simulink model "PEMFuelCellSystem_Before_v01"  (R2025b)
settings: Solver=VariableStepAuto  StartTime=0.0  StopTime=0.1  MaxStep=0.01  RelTol=1e-3  AbsTol=1e-3
model workspace: external: MATLAB File E:\agentwork_pemfc_cEGR_0519\04_Simulink物理网络模型\01_模型\RouteA_GasMixture_Derived\PEMFuelCellSystemWithACustomLibraryParameters.m (data not in the file)
undefined symbols (not defined in the file): anode_tube_D, cathode_tube_D, cegr_valve_max_area, cegr_valve_open_min_area, comp_rpm_TLU, coolant_num_layers, coolant_num_passes, coolant_tube_D, coolant_w_channels, env_p, env_T, env_yH20, env_yO2, radiator_air_area_fins, radiator_air_area_primary, radiator_eta_fin, radiator_N_tubes, radiator_rho, radiator_t_wall, radiator_tube_H, radiator_W, routeA_air_pid_Ki, routeA_air_pid_Kp, routeA_anode_inlet_pressure_MPa_abs, routeA_anode_purge_off_n2_mole_fraction, routeA_anode_purge_on_n2_mole_fraction, routeA_anode_recirculation_base_command, routeA_anode_recirculation_current_gain_A_inv, routeA_anode_rh_setpoint, routeA_cathode_humidifier_gain, routeA_cathode_rh_setpoint, routeA_compressor_cmd_direct, routeA_egr_control_Ki_area, routeA_egr_control_Kp_area, routeA_egr_target_input_mode_id, routeA_egr_valve_actuator_tau, routeA_egr_valve_area_direct, routeA_stack_temperature_set_C, routeA_target_egr_ratio_comp_in, routeA_target_mdot_comp_inlet, routeA_target_oer, routeA_target_p_ca_out_MPa, routeA_voltage_current_max_A, routeA_voltage_current_min_A, routeA_voltage_pi_Ki, routeA_voltage_pi_Kp, stack_area, stack_iL, stack_mea_rho, stack_num_cells, stack_num_channels, stack_t_gdl, stack_t_membrane, stack_w_channels, tank_yH2
libraries: fl_lib x63, FuelCell_lib x53, nesl_utility x42, slpidlib x5
(part 1 of 6)
CloseFcn:
  | try,close(h1_PEMFuelCellSystemWithACustomLibrary),end
  | clear h1_PEMFuelCellSystemWithACustomLibrary
  | try,close(h2_PEMFuelCellSystemWithACustomLibrary),end
  | clear h2_PEMFuelCellSystemWithACustomLibrary
  | try,close(h3_PEMFuelCellSystemWithACustomLibrary),end
  | clear h3_PEMFuelCellSystemWithACustomLibrary
  | try,close(h4_PEMFuelCellSystemWithACustomLibrary),end
  | clear h4_PEMFuelCellSystemWithACustomLibrary
  | try,close(h5_PEMFuelCellSystemWithACustomLibrary),end
  | clear h5_PEMFuelCellSystemWithACustomLibrary
  | try,close(h6_PEMFuelCellSystemWithACustomLibrary),end
  | clear h6_PEMFuelCellSystemWithACustomLibrary
  | 
  | clear tout simlog_PEMFuelCellSystemWithACustomLibrary
Description:
  | PEM Fuel Cell System with a Custom Library
settings Model: Creator=The MathWorks, Inc.  LastModifiedBy=ADMIN
settings SolverCC: AutoScaleAbsTol=off  MaxConsecutiveMinStep=10  AlgebraicLoopSolver=TrustRegion  MaxZcPerStep=1.0
settings DataIOCC: SaveFormat=Array  ReturnWorkspaceOutputs=off
settings DebuggingCC: UnconnectedInputMsg=warning  UnconnectedOutputMsg=warning  UnconnectedLineMsg=warning  SymbolicDimsDataTypeCodeGenerationDiagnostic=none
settings ModelReferenceCC: EnableRefExpFcnMdlSchedulingChecks=on
settings SFSimCC: CustomCodeUndefinedFunction=UseInterfaceOnly
settings RTWCC: GPUComputeCapability=3.5  DLArmComputeVersion=19.05
settings SimscapeCC: SimscapeLogType=all  SimscapeLogSimulationStatistics=on  SimscapeLogName=simlog_PEMFuelCellSystem_GasMixture_cEGR_RouteA_v01  SimscapeLogDataHistory=20000.0

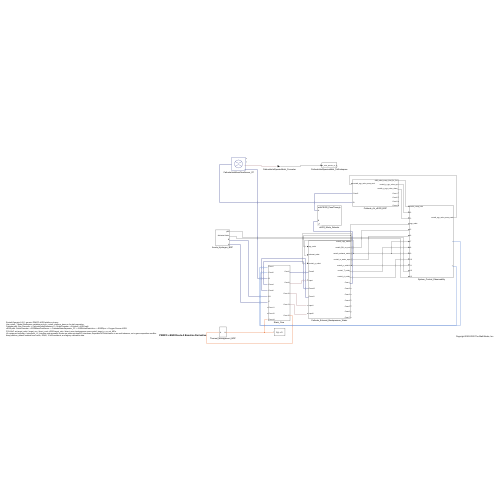
[thumbnail: Simulink's stored preview of the top-level diagram]
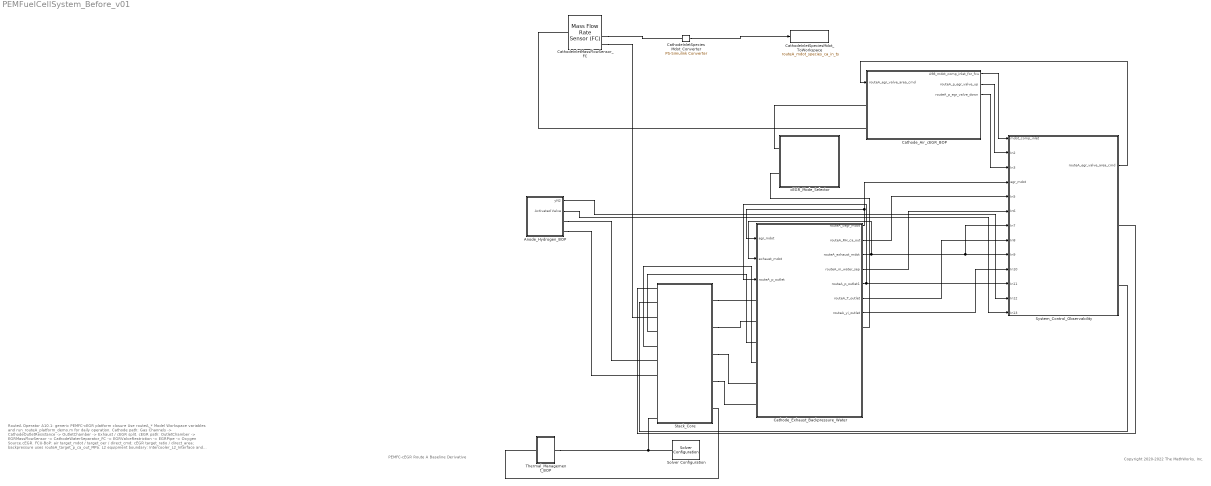
== system PEMFuelCellSystem_Before_v01 ==
  note: PEMFC-cEGR Route A Baseline Derivative
  note: RouteA Operator A10.1: generic PEMFC-cEGR platform closure
      | Use routeA_* Model Workspace variables and run_routeA_platform_demo.m for daily operation.
      | Cathode path: Gas Channels -> CathodeOutletResistance -> OutletChamber -> Exhaust / cEGR split.
      | cEGR path: OutletChamber -> EGRMassFlowSensor -> CathodeWaterSeparator_FC -> EGRValveRestriction -> EGRPipe -> Oxygen Source.cEGR.
      | FCU-BoP: air target_mdot / target_oer / direct_cmd; cEGR target_ratio / direct_area; backpressure uses routeA_target_p_ca_out_MPa.
      | L2 equipment boundary: Intercooler_L2_Interface and separator blocks are pressure-drop/KPI interfaces; SeparatorOrCondensation is an audit observer, not a gas-composition modifier.
      | Keep platform_default isolated from bench, DQ60, 10 kW workbook, and legacy calibration data.
  note: Copyright 2020-2022 The MathWorks, Inc.
  Anode_Hydrogen_BOP : Subsystem
  CathodeInletMassFlowSensor_FC : FuelCell_lib/sensors/Mass Flow Rate Sensor (FC)
      settings: InternalSimscapePortConfiguration="{\"Bottom\":[],\"Left\":[{\"id\":\"A\",\"label\":\"A\",\"type\":\"FuelCell.FuelCell\"}],\"Right\":[{\"id\":\"M\",\"label\":\"M\",\"type\":\"output\"},{\"id\":\"Phi_out\",\"label\":\"Phi\",\"type\":\"output\"},{\"id\":\"M_i\",\"label\":\"M_i\",\"type\":\"output\"},{\"id\":\"B\",\"label\":\"B\",\"type\":\"FuelCell.FuelCell\"}],\"Top\":[]}"
  CathodeInletSpeciesMdot_Converter : nesl_utility/PS-Simulink Converter  PhysicalDomain=network_engine_domain  SubClassName=ps_output  LeftPortType=input  RightPortType=output  PseudoPeriodic=off  Frequencies=[]  VectorFormat=inherit  Unit=inherit  AffineConversion=off
  CathodeInletSpeciesMdot_ToWorkspace : ToWorkspace  VariableName=routeA_mdot_species_ca_in_ts  SaveFormat=Timeseries
  Cathode_Air_cEGR_BOP : Subsystem
  Cathode_Exhaust_Backpressure_Water : Subsystem
  Solver Configuration : nesl_utility/Solver Configuration  PhysicalDomain=network_engine_domain  SubClassName=solver  LeftPortType=input  RightPortType=generic  Tones=[]  Harmonics=[]  SimulateNoise=off  Profile=off  UseLocalSampling=off  EnableSwitchedLinearOptims=on  FrequencyDomain=off  UseCCode=off  RelTol=0.001  AbsTol=1e-06  MinStep=1e-09  ToWorkspace=off  RevertToSquareIcSolve=off  NumHomotopyIterations=100  PhasorMode=off  PhasorModeNumHarmonics=1  ConsistencySolver=NEWTON_XTOL_AFTER_FTOL  IndexReductionMethod=DerivativeReplacement  DoDC=off  ResidualTolerance=1e-09  ConsistencyTolSource=GLOBAL  ConsistencyAbsTol=0.001  ConsistencyRelTol=0.001  ConsistencyTolFactor=0.001  UseLocalSolver=off  LocalSolverChoice=NE_BACKWARD_EULER_ADVANCER  ResolveIndetEquations=on  FunctionEvalNumThread=1  LocalSolverSampleTime=0.001  DoFixedCost=off  MaxNonlinIter=3  MaxModeIter=2  ComputeImpulses=off  ImpulseIterations=2  LinearAlgebra=auto  LinearAlgebraNumThread=0  EquationFormulation=NE_TIME_EF  DelaysMemoryBudget=1024  AutomaticFiltering=on  FilteringTimeConstant=0.001  PartitionStorageMethod=AS_NEEDED  PartitionMemoryBudget=1024  PartitionMethod=ROBUST  MultibodyUseLocalSolver=off  MultibodyLocalSolverChoice=ODE1  MultibodyLocalSolverSampleTime=0.001
  Stack_Core : Subsystem
  System_Control_Observability : Subsystem
  Thermal_Management_BOP : Subsystem
  cEGR_Mode_Selector : Subsystem  Variant=on
  wires:
  CathodeInletSpeciesMdot_Converter/1 -> CathodeInletSpeciesMdot_ToWorkspace/1
  Cathode_Exhaust_Backpressure_Water/5(routeA_p_outlet1) -> System_Control_Observability/11(In11), Cathode_Exhaust_Backpressure_Water/3(routeA_p_outlet)
  Cathode_Exhaust_Backpressure_Water/3(routeA_exhaust_mdot) -> System_Control_Observability/9(In9), System_Control_Observability/7(In7), Cathode_Exhaust_Backpressure_Water/2(exhaust_mdot)
  Cathode_Exhaust_Backpressure_Water/1(routeA_cegr_mdot) -> System_Control_Observability/4(egr_mdot), Cathode_Exhaust_Backpressure_Water/1(egr_mdot)
  Cathode_Air_cEGR_BOP/1(A98_mdot_comp_inlet_for_fcu) -> System_Control_Observability/1(mdot_comp_inlet)
  Cathode_Air_cEGR_BOP/2(routeA_p_egr_valve_up) -> System_Control_Observability/2(In2)
  Cathode_Air_cEGR_BOP/3(routeA_p_egr_valve_down) -> System_Control_Observability/3(In3)
  Cathode_Exhaust_Backpressure_Water/2(routeA_RH_ca_out) -> System_Control_Observability/5(In5)
  Cathode_Exhaust_Backpressure_Water/4(routeA_m_water_sep) -> System_Control_Observability/6(In6)
  Cathode_Exhaust_Backpressure_Water/6(routeA_T_outlet) -> System_Control_Observability/8(In8)
  Cathode_Exhaust_Backpressure_Water/7(routeA_yi_outlet) -> System_Control_Observability/10(In10)
  Anode_Hydrogen_BOP/1(yN2) -> System_Control_Observability/12(In12)
  Anode_Hydrogen_BOP/2(Activated Valve) -> System_Control_Observability/13(In13)
  System_Control_Observability/1(routeA_egr_valve_area_cmd) -> Cathode_Air_cEGR_BOP/1(routeA_egr_valve_area_cmd)
  connections:
  CathodeInletMassFlowSensor_FC/RConn3 -- CathodeInletSpeciesMdot_Converter/LConn1
  CathodeInletMassFlowSensor_FC/RConn4 -- Stack_Core/LConn3
  Cathode_Air_cEGR_BOP/LConn2 -- CathodeInletMassFlowSensor_FC/LConn1
  Stack_Core/RConn1 -- Cathode_Exhaust_Backpressure_Water/LConn1
  Stack_Core/RConn2 -- Cathode_Exhaust_Backpressure_Water/LConn2
  Stack_Core/LConn4 -- Cathode_Exhaust_Backpressure_Water/LConn3
  Stack_Core/LConn5 -- Cathode_Exhaust_Backpressure_Water/LConn4
  Stack_Core/RConn3 -- Cathode_Exhaust_Backpressure_Water/LConn5
  Stack_Core/RConn4 -- Cathode_Exhaust_Backpressure_Water/LConn6
  Anode_Hydrogen_BOP/RConn1 -- Stack_Core/LConn6
  Anode_Hydrogen_BOP/RConn2 -- Stack_Core/LConn7
  Thermal_Management_BOP/RConn1 -- Solver Configuration/RConn1 -- Stack_Core/LConn10
  Thermal_Management_BOP/LConn1 -- Stack_Core/RConn5
  Stack_Core/LConn1 -- System_Control_Observability/RConn1
  Stack_Core/LConn2 -- System_Control_Observability/RConn2
  Cathode_Air_cEGR_BOP/LConn1 -- cEGR_Mode_Selector/LConn1
  cEGR_Mode_Selector/LConn2 -- Cathode_Exhaust_Backpressure_Water/RConn1
